simulink model "SimulinkTask4"  (Simulink 7.8)
settings: Solver=ode45  StartTime=0.0  StopTime=10.0  RelTol=1e-3
values from neighbouring files (symbols this model uses):
  beta = M/sigma/Lr/Ls    (= 6675.56742323)    [initial.m]
  delta = 1/sigma/Ls    (= 7610.14686248)    [initial.m]
  gamma = (Rs+M^2*Rr/Lr^2)/sigma/Ls    (= 173.006113414)    [initial.m]
  J = [0 -1;1 0]    [initial.m]
  M = 0.0005    [initial.m]
undefined symbols (not defined in the file or in its folder): alfa, I, nu
settings Model: Creator=--  LastModifiedBy=--

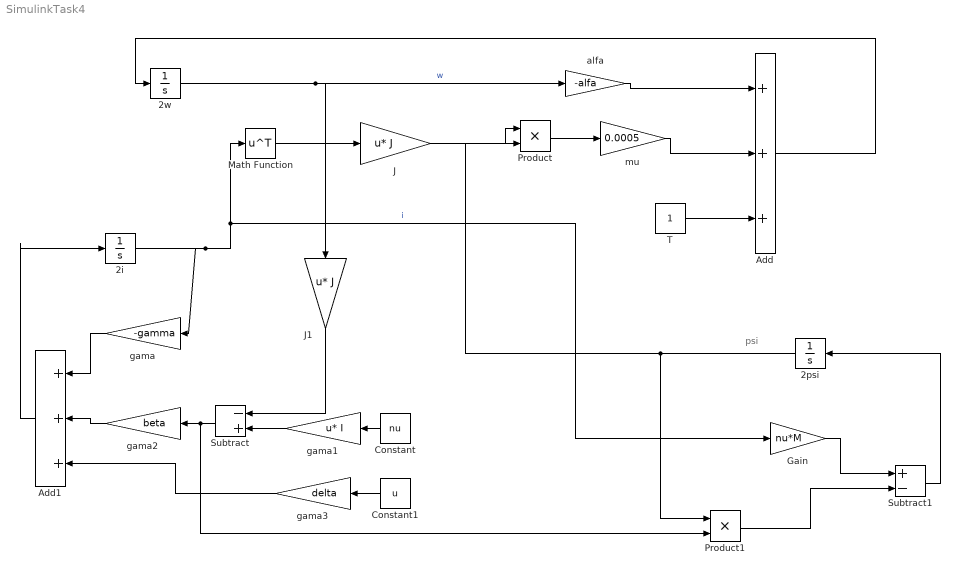
== system SimulinkTask4 ==
  note: psi
  2i : Integrator
  2psi : Integrator
  2w : Integrator
  Add : Sum  Inputs=+++
  Add1 : Sum  Inputs=+++
  Constant : Constant  Value=nu
  Constant1 : Constant  Value=u
  Gain : Gain  Gain=nu*M
  J : Gain  Gain=J  Multiplication=Matrix(u*K)
  J1 : Gain  Gain=J  Multiplication=Matrix(u*K)
  Math Function : Math  Operator=transpose  SaturateOnIntegerOverflow=on
  Product : Product  RndMeth=Zero
  Product1 : Product  RndMeth=Zero
  Subtract : Sum  Inputs=-+
  Subtract1 : Sum  Inputs=+-
  T : Constant
  alfa : Gain  Gain=-alfa
  gama : Gain  Gain=-gamma
  gama1 : Gain  Gain=I  Multiplication=Matrix(u*K)
  gama2 : Gain  Gain=beta
  gama3 : Gain  Gain=delta
  mu : Gain  Gain=0.0005
  wires:
  2w/1 -> alfa/1, J1/1  "w"
  2i/1 -> gama/1, Math Function/1, Gain/1  "i"
  Math Function/1 -> J/1
  J/1 -> Product/1
  2psi/1 -> Product/2, Product1/1
  Product/1 -> mu/1
  T/1 -> Add/3
  mu/1 -> Add/2
  alfa/1 -> Add/1
  Add/1 -> 2w/1
  Constant/1 -> gama1/1
  gama1/1 -> Subtract/2
  J1/1 -> Subtract/1
  Subtract/1 -> gama2/1, Product1/2
  gama/1 -> Add1/1
  gama2/1 -> Add1/2
  Add1/1 -> 2i/1
  Constant1/1 -> gama3/1
  gama3/1 -> Add1/3
  Gain/1 -> Subtract1/1
  Product1/1 -> Subtract1/2
  Subtract1/1 -> 2psi/1
